simulink model "Lab3_original"  (R2020b)
settings: Solver=VariableStepAuto  StartTime=0.0  StopTime=20  MaxStep=1e-3  RelTol=1e-3
libraries: simulink x1
settings Model: Creator=rodsc  LastModifiedBy=rodsc
settings SolverCC: ZeroCrossAlgorithm=Adaptive
settings DebuggingCC: IgnoredZcDiagnostic=none

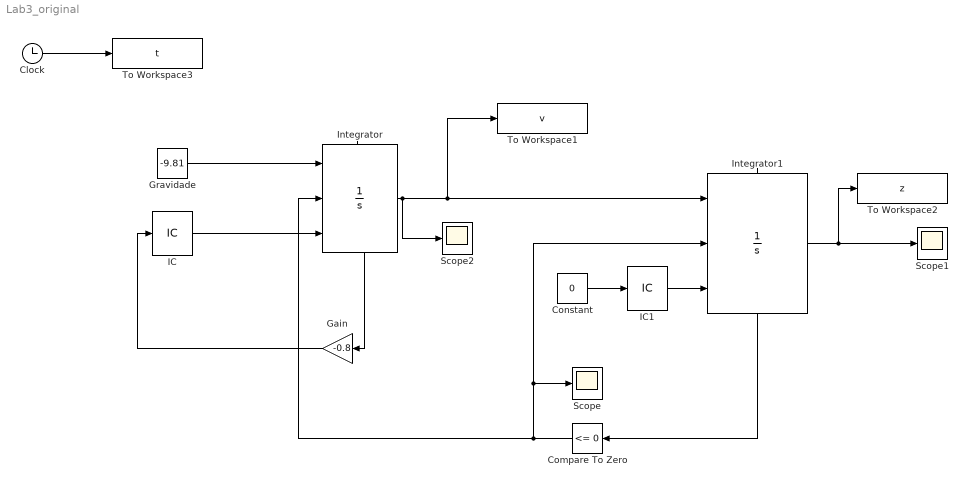
== system Lab3_original ==
  Clock : Clock
  Compare To Zero : simulink/Logic and Bit Operations/Compare To Zero  relop=<=  OutDataTypeStr=boolean
  Constant : Constant  Value=0
  Gain : Gain  Gain=-0.8
  "Gravidade " : Constant  Value=-9.81
  IC : InitialCondition  Value=0
  IC1 : InitialCondition  Value=10
  Integrator : Integrator  ExternalReset=rising  InitialConditionSource=external  ShowStatePort=on
  Integrator1 : Integrator  ExternalReset=rising  InitialConditionSource=external  LowerSaturationLimit=0  ShowStatePort=on
  Scope : Scope
  Scope1 : Scope
  Scope2 : Scope
  To Workspace1 : ToWorkspace  VariableName=v  SampleTime=-1
      settings: Save2DSignal=2-D array (concatenate along first dimension)
  To Workspace2 : ToWorkspace  VariableName=z  SampleTime=-1
      settings: Save2DSignal=2-D array (concatenate along first dimension)
  To Workspace3 : ToWorkspace  VariableName=t  SampleTime=-1
      settings: Save2DSignal=2-D array (concatenate along first dimension)
  wires:
  "Gravidade "/1 -> Integrator/1
  IC/1 -> Integrator/3
  Integrator/1 -> Scope2/1, To Workspace1/1, Integrator1/1
  Gain/1 -> IC/1
  Integrator/State -> Gain/1
  Integrator1/State -> Compare To Zero/1
  Compare To Zero/1 -> Integrator/2, Scope/1, Integrator1/2
  Constant/1 -> IC1/1
  IC1/1 -> Integrator1/3
  Integrator1/1 -> To Workspace2/1, Scope1/1
  Clock/1 -> To Workspace3/1
